simulink model "Schema_X_Q2b"  (R2025b)
settings: Solver=VariableStepAuto  StartTime=0.0  StopTime=10.0  RelTol=1e-3
values from neighbouring files (symbols this model uses):
  g = 9.81    [script_devoir2.m]
  Kdx = -0.367    [script_devoir2.m]
  Kix = -0.176    [script_devoir2.m]
  Kpx = -0.440    (= -0.44)    [script_devoir2.m]
settings Model: Creator=Louis  LastModifiedBy=Louis

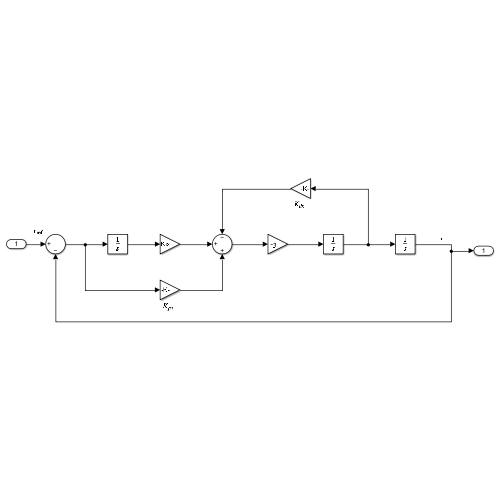
[thumbnail: Simulink's stored preview of the top-level diagram]
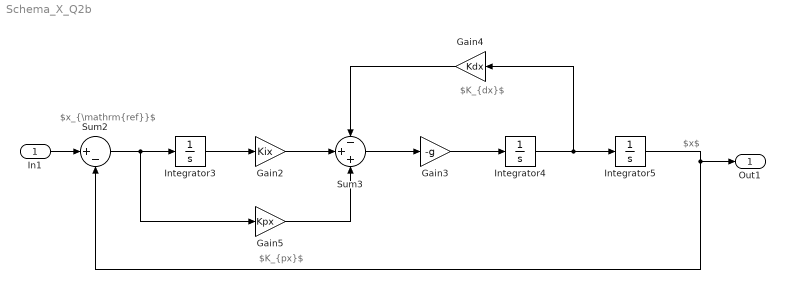
== system Schema_X_Q2b ==
  note: $K_{px}$
  note: $K_{dx}$
  note: $x$
  note: $x_{\mathrm{ref}}$
  In1 : Inport
  Gain2 : Gain  Gain=Kix
  Gain3 : Gain  Gain=-g
  Gain4 : Gain  Gain=Kdx
  Gain5 : Gain  Gain=Kpx
  Integrator3 : Integrator
  Integrator4 : Integrator
  Integrator5 : Integrator
  Sum2 : Sum  Inputs=|+-
  Sum3 : Sum  Inputs=-++
  Out1 : Outport
  wires:
  Gain4/1 -> Sum3/1
  Integrator3/1 -> Gain2/1
  Integrator5/1 -> Out1/1, Sum2/2
  Sum2/1 -> Gain5/1, Integrator3/1
  Gain2/1 -> Sum3/2
  Gain5/1 -> Sum3/3
  Integrator4/1 -> Gain4/1, Integrator5/1
  Sum3/1 -> Gain3/1
  Gain3/1 -> Integrator4/1
  In1/1 -> Sum2/1
